simulink model "model1"  (R2025b)
settings: Solver=VariableStepAuto  StartTime=0.0  StopTime=100  RelTol=1e-3
values from neighbouring files (symbols this model uses):
  A = [0 1; 2 2]    [t_1.m]
  AM = [0 1; -omega0^2 -2*omega0]    [t_1.m]
  B = [0; 8]    [t_1.m]
  B_T = B'    [t_1.m]
  BM = [0; omega0^2]    [t_1.m]
  CM = [1 0]    [t_1.m]
  gamma = gamma_list(j)    [g1_delta0.m]    (also in g1_delta1.m; g2_delta0.m; g2_delta1.m; t_1.m = 500)
  k3_inv = 1 / k3    (= 281.303131129)    [t_1.m]
  P = lyap(AM', Q)    [t_1.m]
  sigma = sigma_list(k)    [g2_delta0.m]    (also in g2_delta1.m; t_1.m = 5)
  x0 = [1;1]    [t_1.m]
settings Model: Creator=eva  LastModifiedBy=eva

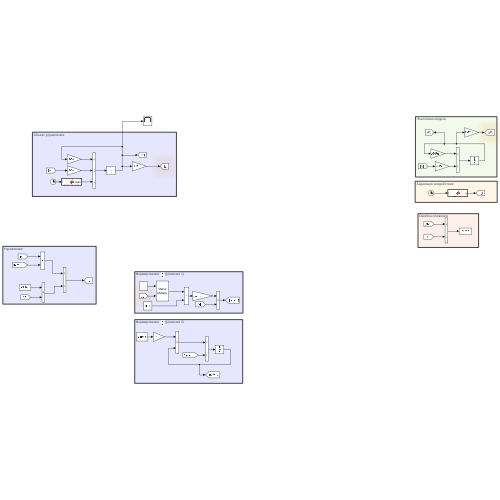
[thumbnail: Simulink's stored preview of the top-level diagram]
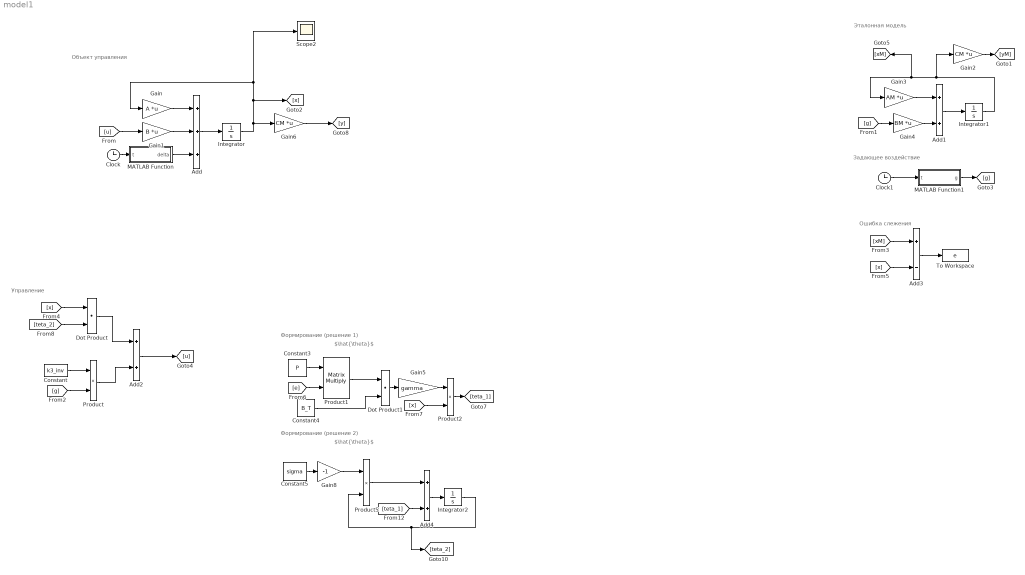
== system model1 ==
  note: $\hat{\theta}$
  note: Формирование (решение 1)
  note: Ошибка слежения
  note: Объект управления
  note: Управление
  note: Задающее воздействие
  note: Эталонная модель
  note: $\hat{\theta}$
  note: Формирование (решение 2)
  Add : Sum  Inputs=+++
  Add1 : Sum
  Add2 : Sum
  Add3 : Sum  Inputs=+-
  Add4 : Sum
  Clock : Clock
  Clock1 : Clock
  Constant : Constant  Value=k3_inv
  Constant3 : Constant  Value=P
  Constant4 : Constant  Value=B_T
  Constant5 : Constant  Value=sigma
  Dot Product : DotProduct  OutDataTypeStr=Inherit: Inherit via internal rule
  Dot Product1 : DotProduct  OutDataTypeStr=Inherit: Inherit via internal rule
  Gain : Gain  Gain=A  Multiplication=Matrix(K*u)
  Gain1 : Gain  Gain=B  Multiplication=Matrix(K*u)
  Gain2 : Gain  Gain=CM  Multiplication=Matrix(K*u)
  Gain3 : Gain  Gain=AM  Multiplication=Matrix(K*u)
  Gain4 : Gain  Gain=BM  Multiplication=Matrix(K*u)
  Gain5 : Gain  Gain=gamma
  Gain6 : Gain  Gain=CM  Multiplication=Matrix(K*u)
  Gain8 : Gain  Gain=-1
  Integrator : Integrator  InitialCondition=x0
  Integrator1 : Integrator  InitialCondition=x0
  Integrator2 : Integrator
  MATLAB Function : MATLAB Function  TreatAsAtomicUnit=on
  MATLAB Function1 : MATLAB Function  TreatAsAtomicUnit=on
  Product : Product
  Product1 : Product  Multiplication=Matrix(*)
  Product2 : Product
  Product5 : Product
  Scope2 : Scope
      settings: ActiveDisplayYMinimum=-93.488546670132735  ActiveDisplayYMaximum=110.28748575630537  DataLoggingVariableName=ScopeData2
  To Workspace : ToWorkspace  VariableName=e  SaveFormat=Timeseries  SampleTime=-1
  wires:
  Gain/1 -> Add/1
  Gain1/1 -> Add/2
  [u] -> Gain1/1
  Add/1 -> Integrator/1
  MATLAB Function/1(delta) -> Add/3
  Clock/1 -> MATLAB Function/1(t)
  Integrator1/1 -> Gain2/1, [xM], Gain3/1
  Add1/1 -> Integrator1/1
  Gain4/1 -> Add1/2
  Gain3/1 -> Add1/1
  Clock1/1 -> MATLAB Function1/1(t)
  MATLAB Function1/1(g) -> [g]
  [g] -> Gain4/1
  [g] -> Product/2
  Product/1 -> Add2/2
  Constant/1 -> Product/1
  Add2/1 -> [u]
  [x] -> Dot Product/1
  [teta_2] -> Dot Product/2
  Dot Product/1 -> Add2/1
  Gain2/1 -> [yM]
  [x] -> Add3/2
  Add3/1 -> To Workspace/1
  Constant3/1 -> Product1/1
  [e] -> Product1/2
  Product1/1 -> Dot Product1/1
  Constant4/1 -> Dot Product1/2
  Dot Product1/1 -> Gain5/1
  Gain5/1 -> Product2/1
  [x] -> Product2/2
  Product2/1 -> [teta_1]
  [xM] -> Add3/1
  Gain6/1 -> [y]
  Integrator/1 -> Scope2/1, Gain/1, [x], Gain6/1
  Constant5/1 -> Gain8/1
  Gain8/1 -> Product5/1
  Product5/1 -> Add4/1
  [teta_1] -> Add4/2
  Add4/1 -> Integrator2/1
  Integrator2/1 -> [teta_2], Product5/2

== matlab function model1/MATLAB Function ==
  data: delta output; t input
function delta = disturbance(t)
    delta = [0.6*sin(10*t) + 0.1*sin(50*t); 
             0.5*cos(12*t) + 0.2*sin(30*t)];
end

== matlab function model1/MATLAB Function1 ==
  data: g output; t input
function g = reference(t)
    g = 2 * sign(sin(t)) + 4;
end
